simulink model "blinkTest"  (R2016b)
settings: Solver=FixedStepDiscrete  StartTime=0.0  StopTime=10  FixedStep=0.001  RelTol=1e-3
settings Model: ExtModeTrigDuration=2  Creator=oelkawok  LastModifiedBy=oelkawok
settings DataIOCC: SaveOutput=off  SaveTime=off
settings OptimizationCC: DefaultParameterBehavior=Inlined  UseFloatMulNetSlope=on  DefaultUnderspecifiedDataType=single  EfficientFloat2IntCast=on  MaxStackSize=64
settings DebuggingCC: ParameterTunabilityLossMsg=error
settings HardwareCC: ProdBitPerInt=16  ProdBitPerPointer=16  ProdBitPerSizeT=16  ProdBitPerPtrDiffT=16  ProdLargestAtomicFloat=None  ProdWordSize=8  ProdHWDeviceType=Atmel->AVR  UseEmbeddedCoderFeatures=off
settings SFSimCC: SimCustomHeaderCode=|
  | #ifndef MATLAB_MEX_FILE
  | #include "../I_O_Wrapper.h"
  | #else
  | #include "I_O_Wrapper.h"
  | #endif
settings RTWCC: SystemTargetFile=ert.tlc  GenerateMakefile=off  TemplateMakefile=RTW.MSVCBuild  Description=Create Visual C/C++ Solution File for Embedded Coder  GenerateReport=on  RTWUseSimCustomCode=on  Toolchain=Arduino AVR  BuildConfiguration=Faster Runs  IncludeHyperlinkInReport=on  LaunchReport=on  GenerateTraceInfo=on  GenerateTraceReport=on  GenerateTraceReportSl=on  GenerateTraceReportSf=on  GenerateTraceReportEml=on
settings RTWCC: CustomHeaderCode=|
  | #ifndef MATLAB_MEX_FILE
  | #include "../I_O_Wrapper.h"
  | #else
  | #include "I_O_Wrapper.h"
  | #endif
settings CodeAppCC: ForceParamTrailComments=on  IgnoreCustomStorageClasses=off  OperatorAnnotations=on  SimulinkDataObjDesc=on  SFDataObjDesc=on  MATLABFcnDesc=on  InsertBlockDesc=on  MATLABSourceComments=on
settings ERTTargetCC: GenerateSampleERTMain=on  InlinedParameterPlacement=NonHierarchical  ERTCustomFileTemplate=example_file_process.tlc

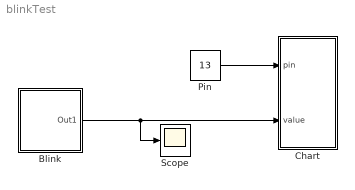
== system blinkTest ==
  Blink : Subsystem  TreatAsAtomicUnit=on
      settings: RTWSystemCode=Nonreusable function  RTWFcnNameOpts=Use subsystem name  RTWFileNameOpts=Use subsystem name  FunctionInterfaceSpec=Allow arguments
  Chart : Stateflow chart  TreatAsAtomicUnit=on
  Pin : Constant  Value=13  OutDataTypeStr=uint8
  Scope : Scope
  wires:
  Blink/1(Out1) -> Scope/1, Chart/2(value)
  Pin/1 -> Chart/1(pin)

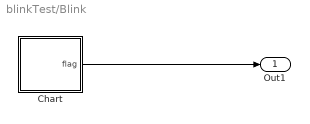
== system blinkTest/Blink ==
  Chart : Stateflow chart  TreatAsAtomicUnit=on
  Out1 : Outport
  wires:
  Chart/1(flag) -> Out1/1

== stateflow chart blinkTest/Chart ==
  (default) -> (junction 1)
  (junction 1) -> (junction 3) : {
      | digitalWrite(pin, value);
      | }
  data: pin input uint8; value input boolean

== stateflow chart blinkTest/Blink/Chart ==
  state on
    en:
    flag = true;
  state off
    en:
    flag = false;
  (default) -> off
  on -> off : [after(1000,tick)]
  off -> on : [after(1000,tick)]
  data: flag output boolean
